simulink model "rocket_landing_part_E"  (R2024b)
settings: Solver=VariableStepAuto  StartTime=0.0  StopTime=10  RelTol=1e-3
model workspace (MAT data in the model file):
  TMAX = 10
  omega0 = '0'
  optobj = 'Minimum time'
  theta0 = '5'
  v0 = '0'
  x0 = '5'
values from neighbouring files (symbols this model uses):
  kd_theta = 1.884    [Systems_Project_Part2e.m]
  kd_x = 3.049    [Systems_Project_Part2e.m]
  kp_theta = 2.217    [Systems_Project_Part2e.m]
  kp_x = 0.7622    [Systems_Project_Part2e.m]
undefined symbols (not defined in the file or in its folder): stop_time, x, X, y, Y, Z
libraries: sm_lib x15, nesl_utility x5, simulink_extras x2, simulink x1
settings Model: Creator=laure  LastModifiedBy=anish
settings RTWCC: GPUComputeCapability=3.5
settings ExplorerConfigSet: InternalSimMechanicsExplorerSettings="<ExplorerConfiguration><canonicalview>default</canonicalview><AnimationSetting><BasePlaybackSpeed>1.0</BasePlaybackSpeed><PlaybackSpeedFactor>1.0</PlaybackSpeedFactor></AnimationSetting><TilePanel><TileInfo><Tiles Columns=\"1\" Count=\"1\" Rows=\"1\"><Column Weight=\"1\"/><Row Weight=\"1\"/><Tile Height=\"1\" Width=\"1\" X=\"0\" Y=\"0\"/></Tiles></TileInfo><SceneInfo><SceneViewer><BGColor><R>0.141176477074623108</R><G>0.341176480054855347</G><B>0.498039215803146362</B></BGColor><Camera><DoPerspective>on</DoPerspective><Position><X>0</X><Y>-800</Y><Z>49</Z></Position><Center><X>0</X><Y>-799</Y><Z>49</Z></Center><Up><X>0</X><Y>0</Y><Z>1</Z></Up><ViewLimDist>1</ViewLimDist><YLim>0.466307658154998583</YLim><XLim>0.681174912402890076</XLim></Camera></SceneViewer></SceneInfo></TilePanel><MechEditorPanel><Cameras><Camera><Id>Camera1</Id><Value><Name>Camera1</Name><NativeCamera><PositionTrackingFeature>Animation.Cam_Frame1.R</PositionTrackingFeature><CenterTrackingFeature>Animation.Cam_Frame1.R</CenterTrackingFeature><UpVectorTrackingFeature>Animation.Cam_Frame1.R</UpVectorTrackingFeature><CenterTrackingOrigin>off</CenterTrackingOrigin><CenterTrackingDirection>+Y</CenterTrackingDirection><UpVectorTrackingDirection>+Z</UpVectorTrackingDirection></NativeCamera></Value></Camera></Cameras><GfxPanelCameraMap><MapElement CameraMLId=\"Camera1\" GfxPanelIndex=\"0\"/></GfxPanelCameraMap><VideoCreator><PlaybackSpeedRatio>1.0</PlaybackSpeedRatio><FrameRate>30</FrameRate><VideoFormat>Uncompressed AVI</VideoFormat><FrameSize>auto</FrameSize></VideoCreator></MechEditorPanel></ExplorerConfiguration>"

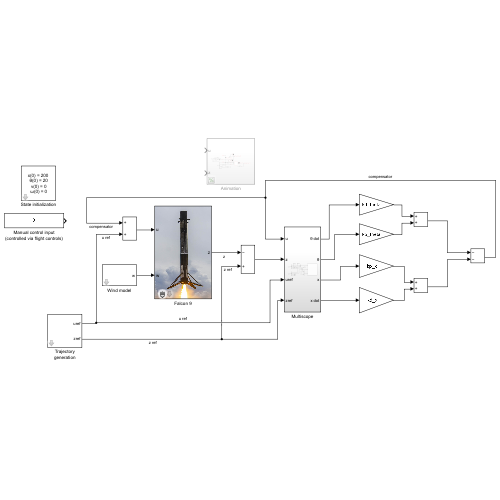
[thumbnail: Simulink's stored preview of the top-level diagram]
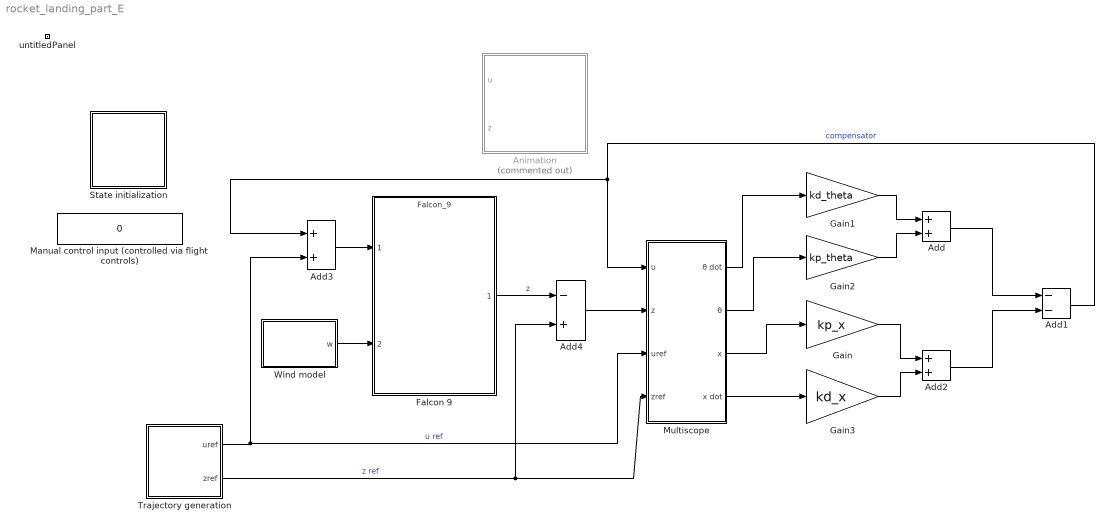
== system rocket_landing_part_E ==
  Add : Sum
  Add1 : Sum  Inputs=--
  Add2 : Sum
  Add3 : Sum
  Add4 : Sum  Inputs=-+
  Animation : Subsystem  Commented=on  InitFcn=|
      | x = linspace(-3000,3000,500);
      | y=x;
      | Z = 1-cos(x*2*pi/3000*2)'*cos(y*2*pi/3000*2);
  Falcon 9 : ModelReference  ModelNameDialog=Falcon_9.slxp  ModelReferenceVersion=1.0  CopyOfModelProtected=on
  Gain : Gain  Gain=kp_x
  Gain1 : Gain  Gain=kd_theta
  Gain2 : Gain  Gain=kp_theta
  Gain3 : Gain  Gain=kd_x
  Manual control input (controlled via flight controls) : Constant  Value=0
  Multiscope : Subsystem
  State initialization : Subsystem  Priority=1  InitFcn=|  mask{x0=200, theta0=20, v0=0, omega0=0}
      | % extract init values, add to model workspace
      | x0 = str2double(get_param(gcb, 'x0'));
      | theta0 = str2double(get_param(gcb, 'theta0'));
      | v0 = str2double(get_param(gcb, 'v0'));
      | omega0 = str2double(get_param(gcb, 'omega0'));
      | 
      | % make z0 tunable from protected Falcon block
      | z0 = Simulink.Parameter;
      | z0.Value = [x0; theta0; v0; omega0];
      | z0.CoderInfo.StorageClass = 'ExportedGlobal';
      | 
      | stop_time = str2double(get_param(bdroot,'StopTime'));
      mask prompts: x0 "horizontal position x(0) (meters):"; theta0 "rotation angle θ(0) (degrees):"; v0 "horizontal velocity v(0) (meters/sec):"; omega0 "angular velocity ω(0) (degrees/sec):"
      mask help: Set the initial values for the rocket
      mask Display:
      | fprintf('x(0) = %s\n θ(0) = %s\n v(0) = %s\n ω(0) = %s',...
      |     get_param(gcb,'x0'), get_param(gcb,'theta0'),...
      |     get_param(gcb,'v0'), get_param(gcb,'omega0'));
      | text(5, 10, 'Gain');
  Trajectory generation : Subsystem  InitFcn=|  mask{optobj=Minimum effort, TMAX=15, umax=15, thetamax=30}
      | % extract selected options and run trajectory generation
      | 
      | optobj = get_param(gcb,'optobj');
      | TMAX = str2double(get_param(gcb, 'TMAX'));
      | umax = str2double(get_param(gcb,'umax'));
      | thetamax = str2double(get_param(gcb,'thetamax'));
      | 
      | [zopt,uopt] = falcon_trajectory_generation(optobj, z0.Value, TMAX, umax, thetamax);
      mask prompts: optobj "Optimization method"; TMAX "Maximum time available (sec)"; umax "Maximum gimbal angle u (deg)"; thetamax "Maximum rocket angle θ (deg)"
      mask help:
      | Minimum time: Attempt to land the rocket as fast as possible while respecting constraints. If this would take longer than the maximum time available, then land as close to the landing pad as possible within the allotted time.
      |
      | Minimum effort: Attempt to land the rocket using as little effort as possible while using all available time. If this is not possible, then land as close to the landing pad as possible within the allotted time.
      mask TypeOptions optobj: Minimum time | Minimum effort
      mask Callback optobj:
      | % this code is executed when a radio button is clicked
      |     % switch get_param(gcb,'optobj')
      |     %     case 'Minimum time'
      |     %         mask_visibilities = get_param(gcb, 'MaskVisibilities');
      |     %         mask_visibilities{4} = 'off';
      |     %         set_param(gcb, 'MaskVisibilities', mask_visibilities);
      |     %     case 'Minimum effort'
      |     %         mask_visibilities = get_param(gcb, 'MaskVisibilities');
      |     %         mask_visibilities{4} = 'on';
      |     %         set_param(gcb, 'MaskVisibilities', mask_visibilities);
      |     % end
  Wind model : Subsystem  mask{wind_type=No wind, wind_strength=10, wind_selector=1}
      mask prompts: wind_type "Wind type"; wind_strength "Wind speed (m/s)"; wind_selector "Wind selector (numerical)"
      mask TypeOptions wind_type: No wind | Constant wind | Variable wind
      mask Callback wind_type:
      | switch get_param(gcb,'wind_type')
      |         case 'No wind'
      |             mask_visibilities = get_param(gcb, 'MaskVisibilities');
      |             mask_visibilities{2} = 'off';
      |             set_param(gcb,'MaskVisibilities', mask_visibilities);
      |             set_param(gcb,'wind_selector','1')
      |         case 'Constant wind'
      |             mask_visibilities = get_param(gcb, 'MaskVisibilities');
      |             mask_visibilities{2} = 'on';
      |             set_param(gcb,'MaskVisibilities', mask_visibilities);
      |             set_param(gcb,'wind_selector','2')
      |         case 'Variable wind'
      |             mask_visibilities = get_param(gcb, 'MaskVisibilities');
      |             mask_visibilities{2} = 'on';
      |             set_param(gcb,'MaskVisibilities', mask_visibilities);
      |             set_param(gcb,'wind_selector','3')
      |     end
  untitledPanel : Subsystem  Tag=HiddenForWebPanel  IsWebBlockPanel=on
  wires:
  Wind model/1(w) -> Falcon 9/2
  Falcon 9/1 -> Add4/1  "z"
  Multiscope/2(θ) -> Gain2/1
  Multiscope/1(θ dot) -> Gain1/1
  Gain1/1 -> Add/1
  Gain2/1 -> Add/2
  Add1/1 -> Add3/1, Multiscope/1(u)  "compensator"
  Multiscope/3(x) -> Gain/1
  Multiscope/4(x dot) -> Gain3/1
  Gain/1 -> Add2/1
  Gain3/1 -> Add2/2
  Add/1 -> Add1/1
  Add2/1 -> Add1/2
  Trajectory generation/1(uref) -> Add3/2, Multiscope/3(uref)  "u ref"
  Trajectory generation/2(zref) -> Add4/2, Multiscope/4(zref)  "z ref"
  Add3/1 -> Falcon 9/1
  Add4/1 -> Multiscope/2(z)

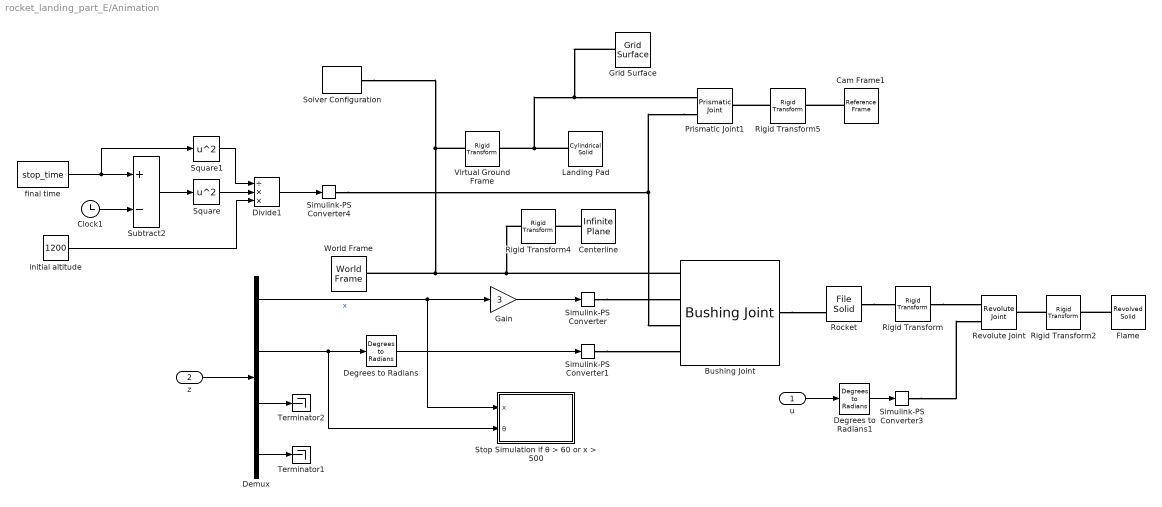
== system rocket_landing_part_E/Animation ==
  u : Inport
  z : Inport  Port=2
  Bushing Joint : sm_lib/Joints/Bushing Joint  JointMode=Normal  CompositeWrenchDir=FollowerOnBase  CompositeWrenchFrame=BaseFrame  SenseConstraintForce=off  SenseConstraintTorque=off  SenseTotalForce=off  SenseTotalTorque=off  PxPositionTargetSpecify=off  PxPositionTargetPriority=High  PxPositionTargetValue=0  PxPositionTargetValueUnits=m  PxVelocityTargetSpecify=off  PxVelocityTargetPriority=High  PxVelocityTargetValue=0  PxVelocityTargetValueUnits=m/s  PxEquilibriumPosition=0  PxEquilibriumPositionUnits=m  PxSpringStiffness=0  PxSpringStiffnessUnits=N/m  PxDampingCoefficient=0  PxDampingCoefficientUnits=N/(m/s)  PxLowerLimitSpecify=off  PxLowerLimitBound=-1  PxLowerLimitBoundUnits=m  PxLowerLimitStiffness=1e6  PxLowerLimitStiffnessUnits=N/m  PxLowerLimitDamping=1e3  PxLowerLimitDampingUnits=N/(m/s)  PxLowerLimitTransitionRegionWidth=1e-4  PxLowerLimitTransitionRegionWidthUnits=m  PxUpperLimitSpecify=off  PxUpperLimitBound=1  PxUpperLimitBoundUnits=m  PxUpperLimitStiffness=1e6  PxUpperLimitStiffnessUnits=N/m  PxUpperLimitDamping=1e3  PxUpperLimitDampingUnits=N/(m/s)  PxUpperLimitTransitionRegionWidth=1e-4  PxUpperLimitTransitionRegionWidthUnits=m  PxTorqueActuationMode=ComputedTorque  PxMotionActuationMode=InputMotion  PxSensePosition=off  PxSenseVelocity=off  PxSenseAcceleration=off  PxSenseTorqueForce=off  PxSenseLowerLimitTorqueForce=off  PxSenseUpperLimitTorqueForce=off  PyPositionTargetSpecify=off  PyPositionTargetPriority=High  PyPositionTargetValue=0  PyPositionTargetValueUnits=m  PyVelocityTargetSpecify=off  PyVelocityTargetPriority=High  PyVelocityTargetValue=0  PyVelocityTargetValueUnits=m/s  PyEquilibriumPosition=0  PyEquilibriumPositionUnits=m  PySpringStiffness=0  PySpringStiffnessUnits=N/m  PyDampingCoefficient=0  PyDampingCoefficientUnits=N/(m/s)  PyLowerLimitSpecify=off  PyLowerLimitBound=-1  PyLowerLimitBoundUnits=m  PyLowerLimitStiffness=1e6  PyLowerLimitStiffnessUnits=N/m  PyLowerLimitDamping=1e3  PyLowerLimitDampingUnits=N/(m/s)  PyLowerLimitTransitionRegionWidth=1e-4  PyLowerLimitTransitionRegionWidthUnits=m  PyUpperLimitSpecify=off  PyUpperLimitBound=1  PyUpperLimitBoundUnits=m  PyUpperLimitStiffness=1e6  PyUpperLimitStiffnessUnits=N/m  PyUpperLimitDamping=1e3  PyUpperLimitDampingUnits=N/(m/s)  PyUpperLimitTransitionRegionWidth=1e-4  PyUpperLimitTransitionRegionWidthUnits=m  PyTorqueActuationMode=NoTorque  PyMotionActuationMode=ComputedMotion  PySensePosition=off  PySenseVelocity=off  PySenseAcceleration=off  PySenseTorqueForce=off  PySenseLowerLimitTorqueForce=off  PySenseUpperLimitTorqueForce=off  PzPositionTargetSpecify=off  PzPositionTargetPriority=High  PzPositionTargetValue=0  PzPositionTargetValueUnits=m  PzVelocityTargetSpecify=off  PzVelocityTargetPriority=High  PzVelocityTargetValue=0  PzVelocityTargetValueUnits=m/s  PzEquilibriumPosition=0  PzEquilibriumPositionUnits=m  PzSpringStiffness=0  PzSpringStiffnessUnits=N/m  PzDampingCoefficient=0  PzDampingCoefficientUnits=N/(m/s)  PzLowerLimitSpecify=off  PzLowerLimitBound=-1  PzLowerLimitBoundUnits=m  PzLowerLimitStiffness=1e6  PzLowerLimitStiffnessUnits=N/m  PzLowerLimitDamping=1e3  PzLowerLimitDampingUnits=N/(m/s)  PzLowerLimitTransitionRegionWidth=1e-4  PzLowerLimitTransitionRegionWidthUnits=m  PzUpperLimitSpecify=off  PzUpperLimitBound=1  PzUpperLimitBoundUnits=m  PzUpperLimitStiffness=1e6  PzUpperLimitStiffnessUnits=N/m  PzUpperLimitDamping=1e3  PzUpperLimitDampingUnits=N/(m/s)  PzUpperLimitTransitionRegionWidth=1e-4  PzUpperLimitTransitionRegionWidthUnits=m  PzTorqueActuationMode=ComputedTorque  PzMotionActuationMode=InputMotion  PzSensePosition=off  PzSenseVelocity=off  PzSenseAcceleration=off  PzSenseTorqueForce=off  PzSenseLowerLimitTorqueForce=off  PzSenseUpperLimitTorqueForce=off  RxPositionTargetSpecify=off  RxPositionTargetPriority=High  RxPositionTargetValue=0  RxPositionTargetValueUnits=deg  RxVelocityTargetSpecify=off  RxVelocityTargetPriority=High  RxVelocityTargetValue=0  RxVelocityTargetValueUnits=deg/s  RxEquilibriumPosition=0  RxEquilibriumPositionUnits=deg  RxSpringStiffness=0  RxSpringStiffnessUnits=N*m/deg  RxDampingCoefficient=0  RxDampingCoefficientUnits=N*m/(deg/s)  RxLowerLimitSpecify=off  RxLowerLimitBound=-90  RxLowerLimitBoundUnits=deg  RxLowerLimitStiffness=1e4  RxLowerLimitStiffnessUnits=N*m/deg  RxLowerLimitDamping=10  RxLowerLimitDampingUnits=N*m/(deg/s)  RxLowerLimitTransitionRegionWidth=0.1  RxLowerLimitTransitionRegionWidthUnits=deg  RxUpperLimitSpecify=off  RxUpperLimitBound=90  RxUpperLimitBoundUnits=deg  RxUpperLimitStiffness=1e4  RxUpperLimitStiffnessUnits=N*m/deg  RxUpperLimitDamping=10  RxUpperLimitDampingUnits=N*m/(deg/s)  RxUpperLimitTransitionRegionWidth=0.1  RxUpperLimitTransitionRegionWidthUnits=deg  RxTorqueActuationMode=NoTorque  RxMotionActuationMode=ComputedMotion  RxSensePosition=off  RxSenseVelocity=off  RxSenseAcceleration=off  RxSenseTorqueForce=off  RxSenseLowerLimitTorqueForce=off  RxSenseUpperLimitTorqueForce=off  RyPositionTargetSpecify=off  RyPositionTargetPriority=High  RyPositionTargetValue=0  RyPositionTargetValueUnits=deg  RyVelocityTargetSpecify=off  RyVelocityTargetPriority=High  RyVelocityTargetValue=0  RyVelocityTargetValueUnits=deg/s  RyEquilibriumPosition=0  RyEquilibriumPositionUnits=deg  RySpringStiffness=0  RySpringStiffnessUnits=N*m/deg  RyDampingCoefficient=0  RyDampingCoefficientUnits=N*m/(deg/s)  RyLowerLimitSpecify=off  RyLowerLimitBound=-90  RyLowerLimitBoundUnits=deg  RyLowerLimitStiffness=1e4  RyLowerLimitStiffnessUnits=N*m/deg  RyLowerLimitDamping=10  RyLowerLimitDampingUnits=N*m/(deg/s)  RyLowerLimitTransitionRegionWidth=0.1  RyLowerLimitTransitionRegionWidthUnits=deg  RyUpperLimitSpecify=off  RyUpperLimitBound=90  RyUpperLimitBoundUnits=deg  RyUpperLimitStiffness=1e4  RyUpperLimitStiffnessUnits=N*m/deg  RyUpperLimitDamping=10  RyUpperLimitDampingUnits=N*m/(deg/s)  RyUpperLimitTransitionRegionWidth=0.1  RyUpperLimitTransitionRegionWidthUnits=deg  RyTorqueActuationMode=ComputedTorque  RyMotionActuationMode=InputMotion  RySensePosition=off  RySenseVelocity=off  RySenseAcceleration=off  RySenseTorqueForce=off  RySenseLowerLimitTorqueForce=off  RySenseUpperLimitTorqueForce=off  RzPositionTargetSpecify=off  RzPositionTargetPriority=High  RzPositionTargetValue=0  RzPositionTargetValueUnits=deg  RzVelocityTargetSpecify=off  RzVelocityTargetPriority=High  RzVelocityTargetValue=0  RzVelocityTargetValueUnits=deg/s  RzEquilibriumPosition=0  RzEquilibriumPositionUnits=deg  RzSpringStiffness=0  RzSpringStiffnessUnits=N*m/deg  RzDampingCoefficient=0  RzDampingCoefficientUnits=N*m/(deg/s)  RzLowerLimitSpecify=off  RzLowerLimitBound=-90  RzLowerLimitBoundUnits=deg  RzLowerLimitStiffness=1e4  RzLowerLimitStiffnessUnits=N*m/deg  RzLowerLimitDamping=10  RzLowerLimitDampingUnits=N*m/(deg/s)  RzLowerLimitTransitionRegionWidth=0.1  RzLowerLimitTransitionRegionWidthUnits=deg  RzUpperLimitSpecify=off  RzUpperLimitBound=90  RzUpperLimitBoundUnits=deg  RzUpperLimitStiffness=1e4  RzUpperLimitStiffnessUnits=N*m/deg  RzUpperLimitDamping=10  RzUpperLimitDampingUnits=N*m/(deg/s)  RzUpperLimitTransitionRegionWidth=0.1  RzUpperLimitTransitionRegionWidthUnits=deg  RzTorqueActuationMode=NoTorque  RzMotionActuationMode=ComputedMotion  RzSensePosition=off  RzSenseVelocity=off  RzSenseAcceleration=off  RzSenseTorqueForce=off  RzSenseLowerLimitTorqueForce=off  RzSenseUpperLimitTorqueForce=off
  Cam Frame1 : sm_lib/Frames and Transforms/Reference Frame
  Centerline : sm_lib/Curves and Surfaces/Infinite Plane  GraphicType=Rectangle  GraphicPlaneWidth=1500  GraphicPlaneWidthUnits=m  GraphicPlaneHeight=1  GraphicPlaneHeightUnits=m  GraphicVisPropType=SimpleVisualProperties  GraphicDiffuseColor=[0 1 0]  GraphicOpacity=1  GraphicSpecularColor=[0.5 0.5 0.5 1.0]  GraphicAmbientColor=[0.15 0.15 0.15 1.0]  GraphicEmissiveColor=[0.0 0.0 0.0 1.0]  GraphicShininess=75
  Clock1 : Clock
  Degrees to Radians : simulink_extras/Transformations/Degrees to Radians
  Degrees to Radians1 : simulink_extras/Transformations/Degrees to Radians
  Demux : Demux
  Divide1 : Product  Inputs=/**
  Flame : sm_lib/Body Elements/Revolved Solid  RevolutionCrossSection=[0 0; 0 -60; 4 -25; 4.2 -20; 4 -15; 2 -5; 0.1 -5; 0.1 0]  RevolutionCrossSectionUnits=m  RevolutionExtent=Full  RevolutionAngle=180  RevolutionAngleUnits=deg  ExportConvexHullGeometry=off  InertiaType=PointMass  BasedOnType=Density  Density=1000  DensityUnits=kg/m^3  Mass=0  MassUnits=kg  CenterOfMass=[0 0 0]  CenterOfMassUnits=m  MomentsOfInertia=[1 1 1]  MomentsOfInertiaUnits=kg*m^2  ProductsOfInertia=[0 0 0]  ProductsOfInertiaUnits=kg*m^2  GraphicType=FromGeometry  MarkerShape=Sphere  MarkerSize=10  GraphicVisPropType=AdvancedVisualProperties  GraphicDiffuseColor=[1, 0.5, 0]  GraphicOpacity=1  GraphicSpecularColor=[0.902 0.902 0.902]  GraphicAmbientColor=[0.5804 0.05098 0.05098]  GraphicEmissiveColor=[0.8588 0.5765 0.2078]  GraphicShininess=100  DoExposeReferenceFrame=on  SerializedFrames=<Frames/>
  Gain : Gain  Gain=3
  Grid Surface : sm_lib/Curves and Surfaces/Grid Surface  XGridVector=x*2  XGridVectorUnits=m  YGridVector=y*2  YGridVectorUnits=m  ZHeights=Z*50  ZHeightsUnits=m  GraphicType=FromGeometry  GraphicVisPropType=AdvancedVisualProperties  GraphicDiffuseColor=[0.05882 0.07843 0.3294]  GraphicOpacity=1  GraphicSpecularColor=[0.05882 0.07843 0.3294]  GraphicAmbientColor=[0.05882 0.07843 0.3294]  GraphicEmissiveColor=[0.0 0.0 0.0 1.0]  GraphicShininess=100
  Landing Pad : sm_lib/Body Elements/Cylindrical Solid  CylinderRadius=100  CylinderRadiusUnits=m  CylinderLength=2  CylinderLengthUnits=m  ExportEntireGeometry=off  InertiaType=CalculateFromGeometry  BasedOnType=Density  Density=1000  DensityUnits=kg/m^3  Mass=1  MassUnits=kg  CenterOfMass=[0 0 0]  CenterOfMassUnits=m  MomentsOfInertia=[1 1 1]  MomentsOfInertiaUnits=kg*m^2  ProductsOfInertia=[0 0 0]  ProductsOfInertiaUnits=kg*m^2  GraphicType=FromGeometry  MarkerShape=Sphere  MarkerSize=10  GraphicVisPropType=SimpleVisualProperties  GraphicDiffuseColor=[0.5804 0.05098 0.05098]  GraphicOpacity=1  GraphicSpecularColor=[0.5 0.5 0.5 1.0]  GraphicAmbientColor=[0.15 0.15 0.15 1.0]  GraphicEmissiveColor=[0.0 0.0 0.0 1.0]  GraphicShininess=75  DoExposeReferenceFrame=on  SerializedFrames=<Frames/>
  Prismatic Joint1 : sm_lib/Joints/Prismatic Joint  JointMode=Normal  CompositeWrenchDir=FollowerOnBase  CompositeWrenchFrame=BaseFrame  SenseConstraintForce=off  SenseConstraintTorque=off  SenseTotalForce=off  SenseTotalTorque=off  PositionTargetSpecify=off  PositionTargetPriority=High  PositionTargetValue=0  PositionTargetValueUnits=m  VelocityTargetSpecify=off  VelocityTargetPriority=High  VelocityTargetValue=0  VelocityTargetValueUnits=m/s  EquilibriumPosition=0  EquilibriumPositionUnits=m  SpringStiffness=0  SpringStiffnessUnits=N/m  DampingCoefficient=0  DampingCoefficientUnits=N/(m/s)  LowerLimitSpecify=off  LowerLimitBound=-1  LowerLimitBoundUnits=m  LowerLimitStiffness=1e6  LowerLimitStiffnessUnits=N/m  LowerLimitDamping=1e3  LowerLimitDampingUnits=N/(m/s)  LowerLimitTransitionRegionWidth=1e-4  LowerLimitTransitionRegionWidthUnits=m  UpperLimitSpecify=off  UpperLimitBound=1  UpperLimitBoundUnits=m  UpperLimitStiffness=1e6  UpperLimitStiffnessUnits=N/m  UpperLimitDamping=1e3  UpperLimitDampingUnits=N/(m/s)  UpperLimitTransitionRegionWidth=1e-4  UpperLimitTransitionRegionWidthUnits=m  TorqueActuationMode=ComputedTorque  MotionActuationMode=InputMotion  SensePosition=off  SenseVelocity=off  SenseAcceleration=off  SenseTorqueForce=off  SenseLowerLimitTorqueForce=off  SenseUpperLimitTorqueForce=off
  Revolute Joint : sm_lib/Joints/Revolute Joint  JointMode=Normal  CompositeWrenchDir=FollowerOnBase  CompositeWrenchFrame=BaseFrame  SenseConstraintForce=off  SenseConstraintTorque=off  SenseTotalForce=off  SenseTotalTorque=off  PositionTargetSpecify=off  PositionTargetPriority=High  PositionTargetValue=0  PositionTargetValueUnits=deg  VelocityTargetSpecify=off  VelocityTargetPriority=High  VelocityTargetValue=0  VelocityTargetValueUnits=deg/s  EquilibriumPosition=0  EquilibriumPositionUnits=deg  SpringStiffness=0  SpringStiffnessUnits=N*m/deg  DampingCoefficient=0  DampingCoefficientUnits=N*m/(deg/s)  LowerLimitSpecify=off  LowerLimitBound=-90  LowerLimitBoundUnits=deg  LowerLimitStiffness=1e4  LowerLimitStiffnessUnits=N*m/deg  LowerLimitDamping=10  LowerLimitDampingUnits=N*m/(deg/s)  LowerLimitTransitionRegionWidth=0.1  LowerLimitTransitionRegionWidthUnits=deg  UpperLimitSpecify=off  UpperLimitBound=90  UpperLimitBoundUnits=deg  UpperLimitStiffness=1e4  UpperLimitStiffnessUnits=N*m/deg  UpperLimitDamping=10  UpperLimitDampingUnits=N*m/(deg/s)  UpperLimitTransitionRegionWidth=0.1  UpperLimitTransitionRegionWidthUnits=deg  TorqueActuationMode=ComputedTorque  MotionActuationMode=InputMotion  SensePosition=off  SenseVelocity=off  SenseAcceleration=off  SenseTorqueForce=off  SenseLowerLimitTorqueForce=off  SenseUpperLimitTorqueForce=off
  Rigid Transform : sm_lib/Frames and Transforms/Rigid Transform  RotationMethod=RotationSequence  FollAlignAxisA=+X  BaseAlignAxisA=+Y  FollAlignAxisB=+Y  BaseAlignAxisB=+Z  RotationStandardAxis=+Z  RotationAngle=0  RotationAngleUnits=deg  RotationArbitraryAxis=[0 0 1]  RotationSequenceAxes=FollowerAxes  RotationSequence=XYX  RotationSequenceAngles=[90 0 0]  RotationSequenceAnglesUnits=deg  RotationMatrix=[1 0 0;0 1 0;0 0 1]  Quaternion=[1 0 0 0]  TranslationMethod=None  TranslationCartesianOffset=[0 0 0]  TranslationCartesianOffsetUnits=m  TranslationStandardAxis=+Z  TranslationStandardOffset=0  TranslationStandardOffsetUnits=m  TranslationROffset=0  TranslationROffsetUnits=m  TranslationThetaOffset=0  TranslationThetaOffsetUnits=deg  TranslationZOffset=0  TranslationZOffsetUnits=m
  Rigid Transform2 : sm_lib/Frames and Transforms/Rigid Transform  RotationMethod=RotationSequence  FollAlignAxisA=+X  BaseAlignAxisA=+Y  FollAlignAxisB=+Y  BaseAlignAxisB=+Z  RotationStandardAxis=+Z  RotationAngle=0  RotationAngleUnits=deg  RotationArbitraryAxis=[0 0 1]  RotationSequenceAxes=FollowerAxes  RotationSequence=XYX  RotationSequenceAngles=[-90 0 0]  RotationSequenceAnglesUnits=deg  RotationMatrix=[1 0 0;0 1 0;0 0 1]  Quaternion=[1 0 0 0]  TranslationMethod=None  TranslationCartesianOffset=[0 0 0]  TranslationCartesianOffsetUnits=m  TranslationStandardAxis=+Z  TranslationStandardOffset=0  TranslationStandardOffsetUnits=m  TranslationROffset=0  TranslationROffsetUnits=m  TranslationThetaOffset=0  TranslationThetaOffsetUnits=deg  TranslationZOffset=0  TranslationZOffsetUnits=m
  Rigid Transform4 : sm_lib/Frames and Transforms/Rigid Transform  RotationMethod=RotationSequence  FollAlignAxisA=+X  BaseAlignAxisA=+Y  FollAlignAxisB=+Y  BaseAlignAxisB=+Z  RotationStandardAxis=+Z  RotationAngle=0  RotationAngleUnits=deg  RotationArbitraryAxis=[0 0 1]  RotationSequenceAxes=FollowerAxes  RotationSequence=XYX  RotationSequenceAngles=[0 90 0]  RotationSequenceAnglesUnits=deg  RotationMatrix=[1 0 0;0 1 0;0 0 1]  Quaternion=[1 0 0 0]  TranslationMethod=Cartesian  TranslationCartesianOffset=[0 0 735]  TranslationCartesianOffsetUnits=m  TranslationStandardAxis=+Z  TranslationStandardOffset=0  TranslationStandardOffsetUnits=m  TranslationROffset=0  TranslationROffsetUnits=m  TranslationThetaOffset=0  TranslationThetaOffsetUnits=deg  TranslationZOffset=0  TranslationZOffsetUnits=m
  Rigid Transform5 : sm_lib/Frames and Transforms/Rigid Transform  RotationMethod=None  FollAlignAxisA=+X  BaseAlignAxisA=+Y  FollAlignAxisB=+Y  BaseAlignAxisB=+Z  RotationStandardAxis=+Z  RotationAngle=0  RotationAngleUnits=deg  RotationArbitraryAxis=[0 0 1]  RotationSequenceAxes=FollowerAxes  RotationSequence=XYX  RotationSequenceAngles=[90 0 0]  RotationSequenceAnglesUnits=deg  RotationMatrix=[1 0 0;0 1 0;0 0 1]  Quaternion=[1 0 0 0]  TranslationMethod=Cartesian  TranslationCartesianOffset=[0 -800 100]  TranslationCartesianOffsetUnits=m  TranslationStandardAxis=+Z  TranslationStandardOffset=0  TranslationStandardOffsetUnits=m  TranslationROffset=0  TranslationROffsetUnits=m  TranslationThetaOffset=0  TranslationThetaOffsetUnits=deg  TranslationZOffset=0  TranslationZOffsetUnits=m
  Rocket : sm_lib/Body Elements/File Solid  ExtGeomFileName=Falcon 9 First Stage v3.stl  UnitType=Custom  ExtGeomFileUnits=m  StepReaderType=HEX  ExportConvexHullGeometry=off  InertiaType=Custom  BasedOnType=DensityFromFile  Density=1000  DensityUnits=kg/m^3  Mass=1  MassUnits=kg  CenterOfMass=[0 0 36]  CenterOfMassUnits=m  MomentsOfInertia=[1 1 1]  MomentsOfInertiaUnits=kg*m^2  ProductsOfInertia=[0 0 0]  ProductsOfInertiaUnits=kg*m^2  GraphicType=FromGeometry  MarkerShape=Sphere  MarkerSize=10  GraphicVisPropType=SimpleVisualProperties  GraphicDiffuseColor=[1.0 1.0 1.0]  GraphicOpacity=1  GraphicSpecularColor=[0.5 0.5 0.5 1.0]  GraphicAmbientColor=[0.15 0.15 0.15 1.0]  GraphicEmissiveColor=[0.0 0.0 0.0 1.0]  GraphicShininess=75  DoExposeReferenceFrame=on  SerializedFrames=<Frames><Frame><Id>Frame2</Id><Value><Name>F2</Name><Origin><Source>ReferenceFrame</Source><FeatureName></FeatureName></Origin><PrimaryAxis><DefinedDirection>+Z</DefinedDirection><Source>ReferenceFrame</Source><SourceDirection>+Z</SourceDirection><FeatureName></FeatureName></PrimaryAxis><SecondaryAxis><DefinedDirection>+X</DefinedDirection><Source>ReferenceFrame</Source><SourceDirection>+X</SourceDirection><FeatureName></FeatureName></SecondaryAxis></Value></Frame><Frame><Id>Frame3</Id><Value><Name>COM</Name><Origin><Source>CenterOfMassFrame</Source><FeatureName></FeatureName></Origin><PrimaryAxis><DefinedDirection>+Z</DefinedDirection><Source>ReferenceFrame</Source><SourceDirection>+Z</SourceDirection><FeatureName></FeatureName></PrimaryAxis><SecondaryAxis><DefinedDirection>+X</DefinedDirection><Source>ReferenceFrame</Source><SourceDirection>+X</SourceDirection><FeatureName></FeatureName></SecondaryAxis></Value></Frame></Frames>
  Simulink-PS Converter{,1,3..4} (4 alike) : nesl_utility/Simulink-PS Converter  PhysicalDomain=network_engine_domain  SubClassName=ps_input  LeftPortType=input  RightPortType=output  PseudoPeriodic=off  Frequencies=[]  NoiseDistribution=none  NoiseParameters=[]  Unit=1  AffineConversion=off  FilteringAndDerivatives=filter  SimscapeFilterOrder=2  InputFilterTimeConstant=0.001  UdotUserProvided=0
  Solver Configuration : nesl_utility/Solver Configuration  PhysicalDomain=network_engine_domain  SubClassName=solver  LeftPortType=input  RightPortType=generic  Tones=[]  Harmonics=[]  SimulateNoise=off  Profile=off  UseLocalSampling=off  EnableSwitchedLinearOptims=on  FrequencyDomain=off  UseCCode=off  RelTol=0.001  AbsTol=0.001  MinStep=1e-09  ToWorkspace=off  RevertToSquareIcSolve=off  NumHomotopyIterations=100  PhasorMode=off  PhasorModeNumHarmonics=1  ConsistencySolver=NEWTON_XTOL_AFTER_FTOL  IndexReductionMethod=DerivativeReplacement  DoDC=off  ResidualTolerance=1e-09  ConsistencyTolSource=GLOBAL  ConsistencyAbsTol=0.001  ConsistencyRelTol=0.001  ConsistencyTolFactor=0.001  UseLocalSolver=off  LocalSolverChoice=NE_BACKWARD_EULER_ADVANCER  ResolveIndetEquations=on  FunctionEvalNumThread=1  LocalSolverSampleTime=0.001  DoFixedCost=off  MaxNonlinIter=3  MaxModeIter=2  ComputeImpulses=off  ImpulseIterations=2  LinearAlgebra=auto  LinearAlgebraNumThread=0  EquationFormulation=NE_TIME_EF  DelaysMemoryBudget=1024  AutomaticFiltering=on  FilteringTimeConstant=0.001  PartitionStorageMethod=AS_NEEDED  PartitionMemoryBudget=1024  PartitionMethod=ROBUST  MultibodyUseLocalSolver=off  MultibodyLocalSolverChoice=ODE1  MultibodyLocalSolverSampleTime=0.001
  Square : Math  Operator=square
  Square1 : Math  Operator=square
  Stop Simulation if θ > 60 or x > 500 : Subsystem
  Subtract2 : Sum  Inputs=+-
  Terminator1 : Terminator
  Terminator2 : Terminator
  Virtual Ground Frame : sm_lib/Frames and Transforms/Rigid Transform  RotationMethod=None  FollAlignAxisA=+X  BaseAlignAxisA=+Y  FollAlignAxisB=+Y  BaseAlignAxisB=+Z  RotationStandardAxis=+Z  RotationAngle=0  RotationAngleUnits=deg  RotationArbitraryAxis=[0 0 1]  RotationSequenceAxes=FollowerAxes  RotationSequence=XYX  RotationSequenceAngles=[0 0 0]  RotationSequenceAnglesUnits=deg  RotationMatrix=[1 0 0;0 1 0;0 0 1]  Quaternion=[1 0 0 0]  TranslationMethod=Cartesian  TranslationCartesianOffset=[0 0 -51]  TranslationCartesianOffsetUnits=m  TranslationStandardAxis=+Z  TranslationStandardOffset=0  TranslationStandardOffsetUnits=m  TranslationROffset=0  TranslationROffsetUnits=m  TranslationThetaOffset=0  TranslationThetaOffsetUnits=deg  TranslationZOffset=0  TranslationZOffsetUnits=m
  World Frame : sm_lib/Frames and Transforms/World Frame
  final time : Constant  Value=stop_time
  initial altitude : Constant  Value=1200
  wires:
  Degrees to Radians/1 -> Simulink-PS Converter1/1
  Degrees to Radians1/1 -> Simulink-PS Converter3/1
  Demux/3 -> Terminator2/1
  Divide1/1 -> Simulink-PS Converter4/1
  initial altitude/1 -> Divide1/3
  z/1 -> Demux/1
  Demux/4 -> Terminator1/1
  Square1/1 -> Divide1/1
  u/1 -> Degrees to Radians1/1
  Gain/1 -> Simulink-PS Converter/1
  Subtract2/1 -> Square/1
  Clock1/1 -> Subtract2/2
  Demux/2 -> Stop Simulation if θ > 60 or x > 500/2(θ), Degrees to Radians/1
  Demux/1 -> Stop Simulation if θ > 60 or x > 500/1(x), Gain/1  "x"
  final time/1 -> Square1/1, Subtract2/1
  Square/1 -> Divide1/2
  connections:
  World Frame/RConn1 -- Rigid Transform4/LConn1 -- Bushing Joint/LConn1 -- Solver Configuration/RConn1 -- Virtual Ground Frame/LConn1
  Prismatic Joint1/LConn2 -- Bushing Joint/LConn3 -- Simulink-PS Converter4/RConn1
  Landing Pad/RConn1 -- Prismatic Joint1/LConn1 -- Grid Surface/LConn1 -- Virtual Ground Frame/RConn1
  Simulink-PS Converter1/RConn1 -- Bushing Joint/LConn4
  Cam Frame1/RConn1 -- Rigid Transform5/RConn1
  Rigid Transform5/LConn1 -- Prismatic Joint1/RConn1
  Rigid Transform/RConn1 -- Revolute Joint/LConn1
  Flame/RConn1 -- Rigid Transform2/RConn1
  Bushing Joint/RConn1 -- Rocket/LConn2
  Simulink-PS Converter/RConn1 -- Bushing Joint/LConn2
  Rigid Transform2/LConn1 -- Revolute Joint/RConn1
  Simulink-PS Converter3/RConn1 -- Revolute Joint/LConn2
  Centerline/LConn1 -- Rigid Transform4/RConn1
  Rocket/RConn1 -- Rigid Transform/LConn1

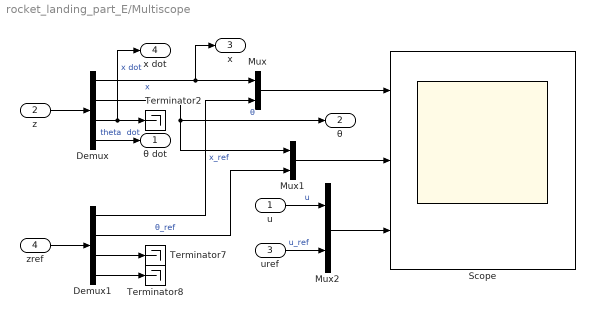
== system rocket_landing_part_E/Multiscope ==
  u : Inport
  z : Inport  Port=2
  uref : Inport  Port=3
  zref : Inport  Port=4
  Demux : Demux
  Demux1 : Demux
  Mux : Mux  Inputs=2
  Mux1 : Mux  Inputs=2
  Mux2 : Mux  Inputs=2
  Scope : Scope  NumInputPorts=3
  Terminator2 : Terminator
  Terminator7 : Terminator
  Terminator8 : Terminator
  θ dot : Outport
  θ : Outport  Port=2
  x : Outport  Port=3
  x dot : Outport  Port=4
  wires:
  z/1 -> Demux/1
  Demux/1 -> x/1, Mux/1  "x"
  Demux/2 -> θ/1, Mux1/1  "θ"
  Demux/3 -> x dot/1, Terminator2/1  "x dot"
  Demux/4 -> θ dot/1  "theta  dot"
  u/1 -> Mux2/1  "u"
  uref/1 -> Mux2/2  "u_ref"
  Demux1/4 -> Terminator8/1
  Demux1/3 -> Terminator7/1
  Demux1/2 -> Mux1/2  "θ_ref"
  Demux1/1 -> Mux/2  "x_ref"
  zref/1 -> Demux1/1
  Mux/1 -> Scope/1
  Mux1/1 -> Scope/2
  Mux2/1 -> Scope/3

== system rocket_landing_part_E/State initialization ==

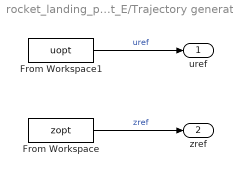
== system rocket_landing_part_E/Trajectory generation ==
  From Workspace : FromWorkspace  VariableName=zopt  OutputAfterFinalValue=Holding final value
  From Workspace1 : FromWorkspace  VariableName=uopt  OutputAfterFinalValue=Setting to zero
  uref : Outport
  zref : Outport  Port=2
  wires:
  From Workspace1/1 -> uref/1  "uref"
  From Workspace/1 -> zref/1  "zref"

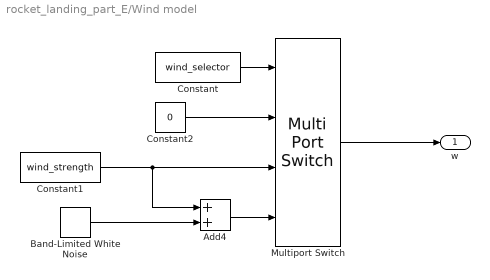
== system rocket_landing_part_E/Wind model ==
  Add4 : Sum
  Band-Limited White Noise : simulink/Sources/Band-Limited White Noise  Cov=0.003 * wind_strength^2  Ts=0.1  seed=[23341]
  Constant : Constant  Value=wind_selector
  Constant1 : Constant  Value=wind_strength
  Constant2 : Constant  Value=0
  Multiport Switch : MultiPortSwitch  SaturateOnIntegerOverflow=off  InputSameDT=off
  w : Outport
  wires:
  Constant/1 -> Multiport Switch/1
  Constant1/1 -> Add4/1, Multiport Switch/3
  Multiport Switch/1 -> w/1
  Constant2/1 -> Multiport Switch/2
  Add4/1 -> Multiport Switch/4
  Band-Limited White Noise/1 -> Add4/2

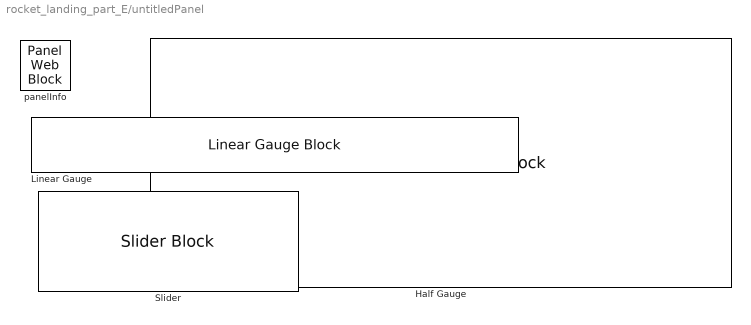
== system rocket_landing_part_E/untitledPanel ==
  Half Gauge : SemiCircularGaugeBlock  Tag=HiddenForWebPanel  PanelInfo="{\"height\":197,\"left\":40,\"panelId\":\"panelId-428ec6e3-ed16-4472-9313-660379ab484c\",\"top\":5,\"type\":\"panelChild\",\"version\":\"2019b\",\"width\":397,\"zIndex\":1500008}"  LabelPosition=Hide  ScaleMin=-90  ScaleMax=90  TickInterval=15
  Linear Gauge : LinearGaugeBlock  Tag=HiddenForWebPanel  PanelInfo="{\"height\":54,\"left\":6,\"panelId\":\"panelId-428ec6e3-ed16-4472-9313-660379ab484c\",\"top\":207,\"type\":\"panelChild\",\"version\":\"2019b\",\"width\":461,\"zIndex\":1500004}"  LabelPosition=Hide  ScaleMin=-200  ScaleMax=200  TickInterval=20
  Slider : SliderBlock  Tag=HiddenForWebPanel  PanelInfo="{\"height\":50,\"left\":120,\"panelId\":\"panelId-428ec6e3-ed16-4472-9313-660379ab484c\",\"top\":273,\"type\":\"panelChild\",\"version\":\"2019b\",\"width\":238,\"zIndex\":1500006}"  LabelPosition=Hide  ScaleMin=-15  ScaleMax=15  TickInterval=5
  panelInfo : PanelWebBlock  Tag=HiddenForWebPanel  PanelInfo="{\"compacted\":false,\"height\":325,\"isActiveTab\":true,\"labels\":{},\"left\":840,\"name\":\"Flight controls\",\"panelId\":\"panelId-428ec6e3-ed16-4472-9313-660379ab484c\",\"popoutData\":{\"height\":370,\"left\":8,\"maximized\":false,\"top\":8,\"width\":494},\"popoutMode\":\"windowHidden\",\"tabIndex\":0,\"tabbedSetId\":\"tabbedSet7084548839\",\"top\":60,\"type\":\"panel\",\"version\":\"2019b\",\"visible\":true,\"width\":469,\"zIndex\":1500002}"  PanelSnapshot=<binary blob, 54332 chars, not shown>

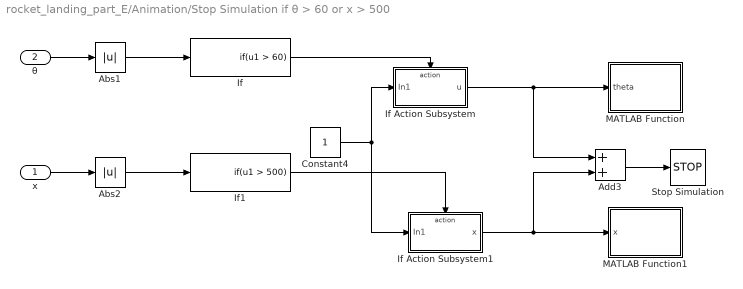
== system rocket_landing_part_E/Animation/Stop Simulation if θ > 60 or x > 500 ==
  x : Inport
  θ : Inport  Port=2
  Abs1 : Abs  SaturateOnIntegerOverflow=off
  Abs2 : Abs  SaturateOnIntegerOverflow=off
  Add3 : Sum
  Constant4 : Constant
  If : If  IfExpression=u1 > 60  ShowElse=off
  If Action Subsystem : Subsystem  TreatAsAtomicUnit=on
  If Action Subsystem1 : Subsystem  TreatAsAtomicUnit=on
  If1 : If  IfExpression=u1 > 500  ShowElse=off
  MATLAB Function : MATLAB Function  TreatAsAtomicUnit=on
  MATLAB Function1 : MATLAB Function  TreatAsAtomicUnit=on
  Stop Simulation : Stop
  wires:
  If/1 -> If Action Subsystem/Action
  Add3/1 -> Stop Simulation/1
  If Action Subsystem/1(u) -> MATLAB Function/1(theta), Add3/1
  Abs1/1 -> If/1
  If1/1 -> If Action Subsystem1/Action
  Constant4/1 -> If Action Subsystem1/1(In1), If Action Subsystem/1(In1)
  If Action Subsystem1/1(x) -> MATLAB Function1/1(x), Add3/2
  Abs2/1 -> If1/1
  x/1 -> Abs2/1
  θ/1 -> Abs1/1

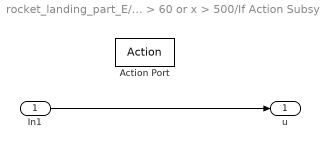
== system rocket_landing_part_E/Animation/Stop Simulation if θ > 60 or x > 500/If Action Subsystem ==
  In1 : Inport
  Action Port : ActionPort  ActionPortLabel=if(u1 > 60)
  u : Outport
  wires:
  In1/1 -> u/1

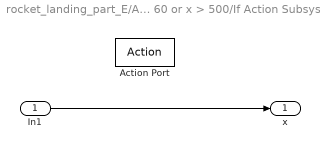
== system rocket_landing_part_E/Animation/Stop Simulation if θ > 60 or x > 500/If Action Subsystem1 ==
  In1 : Inport
  Action Port : ActionPort  ActionPortLabel=if(u1 > 500)
  x : Outport
  wires:
  In1/1 -> x/1

== matlab function rocket_landing_part_E/Animation/Stop Simulation if θ > 60 or x > 500/MATLAB Function ==
  data: theta input
function check_theta(theta)
if theta == 1
    disp('*** Booster Reentry Failed: Angle Too Steep! ***');
    disp('Abort Landing Procedure – Critical Tilt Detected! (Max Angle 60°)');
end

== matlab function rocket_landing_part_E/Animation/Stop Simulation if θ > 60 or x > 500/MATLAB Function1 ==
  data: x input
function check_disp(x)
if x == 1
    fprintf('*** Booster Reentry Failed: Out of Landing Zone! ***\n');
    fprintf('Abort Landing Procedure – Horizontal Deviation Exceeds 500 m!\n');
end
